simulink model "us_capital_nonlinear_1o_simulation_simu"  (R2022b)
settings: Solver=FixedStepAuto  StartTime=0.0  StopTime=N*time_step  FixedStep=5  RelTol=1e-3
values from neighbouring files (symbols this model uses):
  A = temp.A    [us_capital_nonlinear_1o_simulation.m]    (also in us_capital_nonlinear_1o_simulation_data.mat = 1)
  B = temp.B    [us_capital_nonlinear_1o_simulation.m]    (also in us_capital_nonlinear_1o_simulation_data.mat = [0.0303169343876 0.0303169343876 0.0303169343876 -0.03031693)
  C = temp.C    [us_capital_nonlinear_1o_simulation.m]    (also in us_capital_nonlinear_1o_simulation_data.mat = 0.0625)
  D = temp.D    [us_capital_nonlinear_1o_simulation.m]    (also in us_capital_nonlinear_1o_simulation_data.mat = [-0.00381956555672 0.0785006000312 0.00178670572278 -0.00040)
  ds_delay = taud(end)    [us_capital_nonlinear_1o_simulation.m]    (also in us_capital_nonlinear_1o_simulation_data.mat = 41)
settings Model: Creator=chuan  LastModifiedBy=chuan

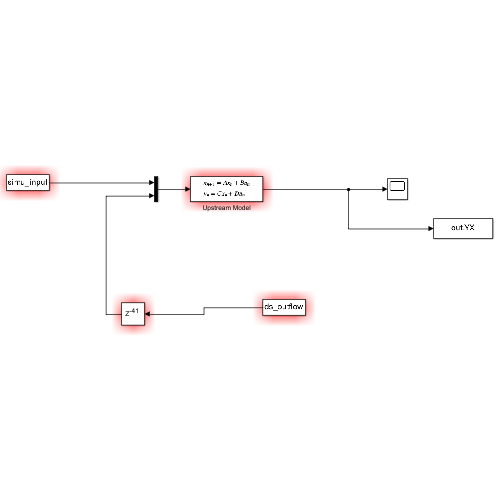
[thumbnail: Simulink's stored preview of the top-level diagram]
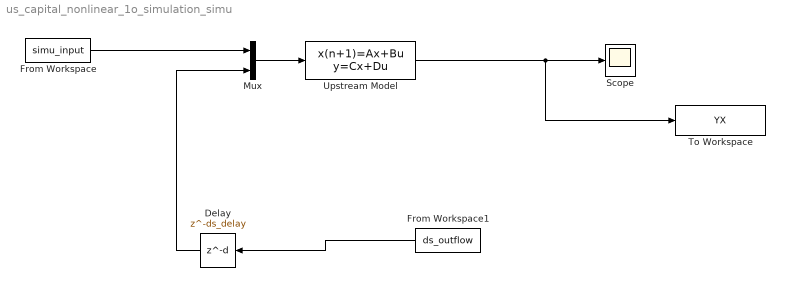
== system us_capital_nonlinear_1o_simulation_simu ==
  Delay : Delay  DelayLength=ds_delay  InitialCondition=0
  From Workspace : FromWorkspace  VariableName=simu_input  SampleTime=-1
  From Workspace1 : FromWorkspace  VariableName=ds_outflow  SampleTime=-1
  Mux : Mux  Inputs=2
  Scope : Scope
  To Workspace : ToWorkspace  VariableName=YX  SaveFormat=Timeseries  SampleTime=-1
  Upstream Model : DiscreteStateSpace  A=A  B=B  C=C  D=D  SampleTime=-1
  wires:
  Upstream Model/1 -> To Workspace/1, Scope/1
  Mux/1 -> Upstream Model/1
  From Workspace/1 -> Mux/1
  From Workspace1/1 -> Delay/1
  Delay/1 -> Mux/2
